simulink model "control_mimo_simulink_Clase10"  (R2019b)
settings: Solver=ode45  StartTime=0.0  StopTime=7  MaxStep=0.01  RelTol=1e-3
values from neighbouring files (symbols this model uses):
  A = [-0.005509 0 0 -0.1588 ... (first row only)    [controlador_mimo_Clase10.m]
  B = [0.28 0 -0.01348 0 ... (first row only)    [controlador_mimo_Clase10.m]
  C = [14.21 0 0 0 ... (first row only)    [controlador_mimo_Clase10.m]
  D = [0 0 0 0 ... (first row only)    [controlador_mimo_Clase10.m]
  xini = 0*[0.2; 0.3; 0; -0.2]    [controlador_mimo_Clase10.m]
undefined symbols (not defined in the file or in its folder): AL, BL, CL, DL, u10, u20, u30, x10n, x20n, x30n
libraries: cstblocks x16
settings Model: Creator=B13  LastModifiedBy=l53

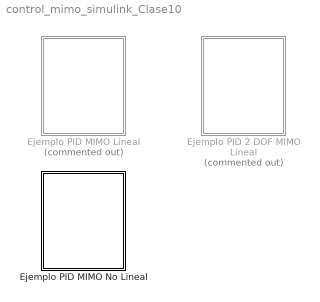
== system control_mimo_simulink_Clase10 ==
  Ejemplo PID 2 DOF MIMO Lineal : Subsystem  Commented=on
  Ejemplo PID MIMO Lineal : Subsystem  Commented=on
  Ejemplo PID MIMO No Lineal : Subsystem

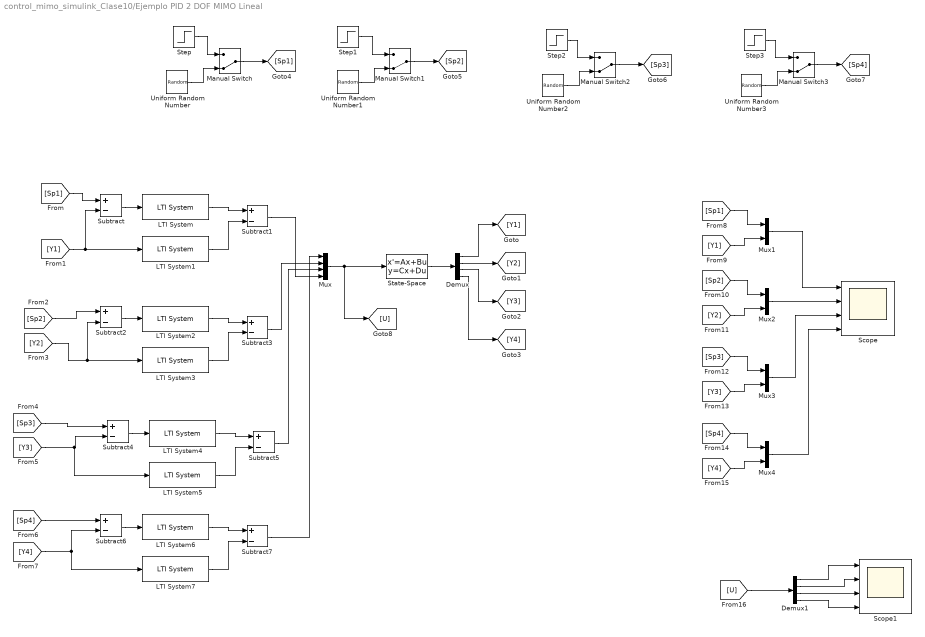
== system control_mimo_simulink_Clase10/Ejemplo PID 2 DOF MIMO Lineal ==
  Demux : Demux
  Demux1 : Demux
  LTI System : cstblocks/LTI System  sys=C14a  IC=[]
  LTI System1 : cstblocks/LTI System  sys=C14b  IC=[]
  LTI System2 : cstblocks/LTI System  sys=C22a  IC=[]
  LTI System3 : cstblocks/LTI System  sys=C22b  IC=[]
  LTI System4 : cstblocks/LTI System  sys=C33a  IC=[]
  LTI System5 : cstblocks/LTI System  sys=C33b  IC=[]
  LTI System6 : cstblocks/LTI System  sys=C41a  IC=[]
  LTI System7 : cstblocks/LTI System  sys=C41b  IC=[]
  Manual Switch{,1..3} (4 alike) : ManualSwitch  CurrentSetting=0
  Mux : Mux
  Mux{1..4} (4 alike) : Mux  Inputs=2
  Scope : Scope  NumInputPorts=4
  Scope1 : Scope  NumInputPorts=4
  State-Space : StateSpace  A=A  B=B  C=C  D=D  InitialCondition=xini
  Step : Step  Time=0  After=0  SampleTime=0
  Step1 : Step  Time=0  After=0  SampleTime=0
  Step2 : Step  Time=0  After=0  SampleTime=0
  Step3 : Step  Time=0  SampleTime=0
  Subtract{,1..7} (8 alike) : Sum  Inputs=+-
  Uniform Random Number : UniformRandomNumber  SampleTime=800
  Uniform Random Number1 : UniformRandomNumber  SampleTime=1000
  Uniform Random Number2 : UniformRandomNumber  SampleTime=1200
  Uniform Random Number3 : UniformRandomNumber  SampleTime=1500
  wires:
  Mux2/1 -> Scope/2
  Step1/1 -> Manual Switch1/1
  Manual Switch/1 -> [Sp1]
  [U] -> Demux1/1
  Step2/1 -> Manual Switch2/1
  [Sp2] -> Mux2/1
  Uniform Random Number/1 -> Manual Switch/2
  [Y3] -> Mux3/2
  Demux/4 -> [Y4]
  Mux/1 -> [U], State-Space/1
  Step3/1 -> Manual Switch3/1
  Manual Switch2/1 -> [Sp3]
  Manual Switch1/1 -> [Sp2]
  Manual Switch3/1 -> [Sp4]
  Mux3/1 -> Scope/3
  Uniform Random Number2/1 -> Manual Switch2/2
  Uniform Random Number3/1 -> Manual Switch3/2
  Uniform Random Number1/1 -> Manual Switch1/2
  Step/1 -> Manual Switch/1
  Demux/2 -> [Y2]
  [Y4] -> Mux4/2
  [Sp1] -> Mux1/1
  [Sp4] -> Mux4/1
  Demux/3 -> [Y3]
  State-Space/1 -> Demux/1
  Demux/1 -> [Y1]
  Demux1/3 -> Scope1/3
  Demux1/1 -> Scope1/1
  Demux1/4 -> Scope1/4
  [Sp3] -> Mux3/1
  [Y1] -> Mux1/2
  Mux1/1 -> Scope/1
  Mux4/1 -> Scope/4
  [Y2] -> Mux2/2
  Demux1/2 -> Scope1/2
  [Sp1] -> Subtract/1
  [Y1] -> Subtract/2, LTI System1/1
  Subtract/1 -> LTI System/1
  LTI System/1 -> Subtract1/1
  LTI System1/1 -> Subtract1/2
  Subtract1/1 -> Mux/4
  [Y2] -> Subtract2/2, LTI System3/1
  [Sp2] -> Subtract2/1
  LTI System3/1 -> Subtract3/2
  LTI System2/1 -> Subtract3/1
  Subtract2/1 -> LTI System2/1
  Subtract3/1 -> Mux/2
  [Sp3] -> Subtract4/1
  LTI System5/1 -> Subtract5/2
  LTI System4/1 -> Subtract5/1
  Subtract4/1 -> LTI System4/1
  [Y3] -> LTI System5/1, Subtract4/2
  Subtract5/1 -> Mux/3
  [Sp4] -> Subtract6/1
  LTI System7/1 -> Subtract7/2
  LTI System6/1 -> Subtract7/1
  Subtract6/1 -> LTI System6/1
  [Y4] -> Subtract6/2, LTI System7/1
  Subtract7/1 -> Mux/1

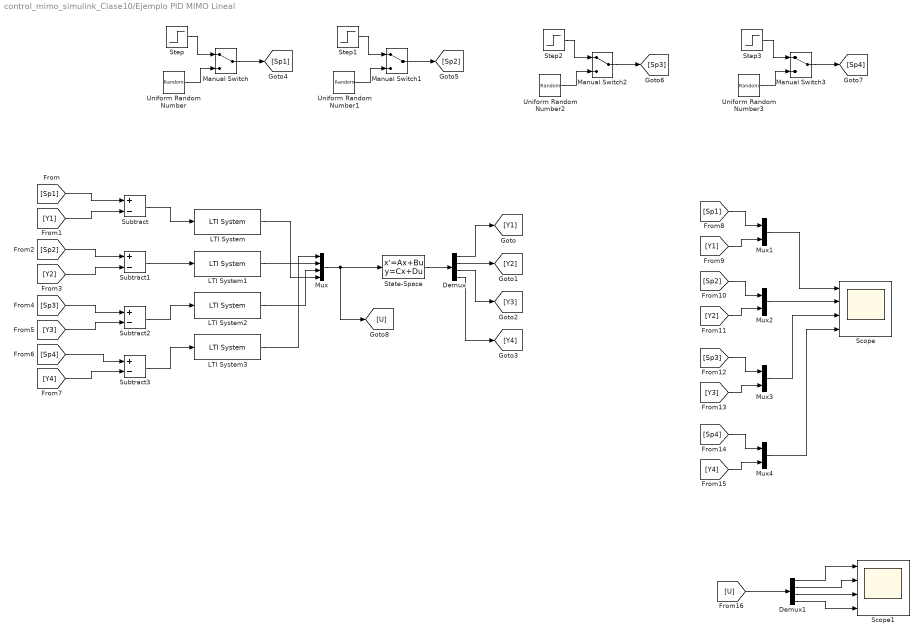
== system control_mimo_simulink_Clase10/Ejemplo PID MIMO Lineal ==
  Demux : Demux
  Demux1 : Demux
  LTI System : cstblocks/LTI System  sys=C14  IC=[]
  LTI System1 : cstblocks/LTI System  sys=C22  IC=[]
  LTI System2 : cstblocks/LTI System  sys=C33  IC=[]
  LTI System3 : cstblocks/LTI System  sys=C41  IC=[]
  Manual Switch{,1..3} (4 alike) : ManualSwitch
  Mux : Mux
  Mux{1..4} (4 alike) : Mux  Inputs=2
  Scope : Scope  NumInputPorts=4
  Scope1 : Scope  NumInputPorts=4
  State-Space : StateSpace  A=A  B=B  C=C  D=D  InitialCondition=xini
  Step{,1..3} (4 alike) : Step  Time=0  After=0  SampleTime=0
  Subtract{,1..3} (4 alike) : Sum  Inputs=+-
  Uniform Random Number : UniformRandomNumber  SampleTime=500
  Uniform Random Number1 : UniformRandomNumber  SampleTime=700
  Uniform Random Number2 : UniformRandomNumber  SampleTime=900
  Uniform Random Number3 : UniformRandomNumber  SampleTime=1100
  wires:
  Mux2/1 -> Scope/2
  Step1/1 -> Manual Switch1/1
  Manual Switch/1 -> [Sp1]
  [Y1] -> Subtract/2
  [U] -> Demux1/1
  LTI System/1 -> Mux/4
  Step2/1 -> Manual Switch2/1
  [Sp2] -> Mux2/1
  Uniform Random Number/1 -> Manual Switch/2
  [Y3] -> Mux3/2
  Demux/4 -> [Y4]
  Mux/1 -> [U], State-Space/1
  Step3/1 -> Manual Switch3/1
  Subtract2/1 -> LTI System2/1
  LTI System1/1 -> Mux/2
  Manual Switch2/1 -> [Sp3]
  Manual Switch1/1 -> [Sp2]
  Subtract3/1 -> LTI System3/1
  Manual Switch3/1 -> [Sp4]
  Mux3/1 -> Scope/3
  Subtract1/1 -> LTI System1/1
  Uniform Random Number2/1 -> Manual Switch2/2
  Uniform Random Number3/1 -> Manual Switch3/2
  Uniform Random Number1/1 -> Manual Switch1/2
  Step/1 -> Manual Switch/1
  [Y3] -> Subtract2/2
  [Sp1] -> Subtract/1
  Demux/2 -> [Y2]
  [Y4] -> Mux4/2
  [Sp1] -> Mux1/1
  LTI System2/1 -> Mux/3
  [Sp4] -> Mux4/1
  [Y2] -> Subtract1/2
  [Sp2] -> Subtract1/1
  Demux/3 -> [Y3]
  [Sp3] -> Subtract2/1
  Subtract/1 -> LTI System/1
  [Sp4] -> Subtract3/1
  State-Space/1 -> Demux/1
  LTI System3/1 -> Mux/1
  [Y4] -> Subtract3/2
  Demux/1 -> [Y1]
  Demux1/3 -> Scope1/3
  Demux1/1 -> Scope1/1
  Demux1/4 -> Scope1/4
  [Sp3] -> Mux3/1
  [Y1] -> Mux1/2
  Mux1/1 -> Scope/1
  Mux4/1 -> Scope/4
  [Y2] -> Mux2/2
  Demux1/2 -> Scope1/2

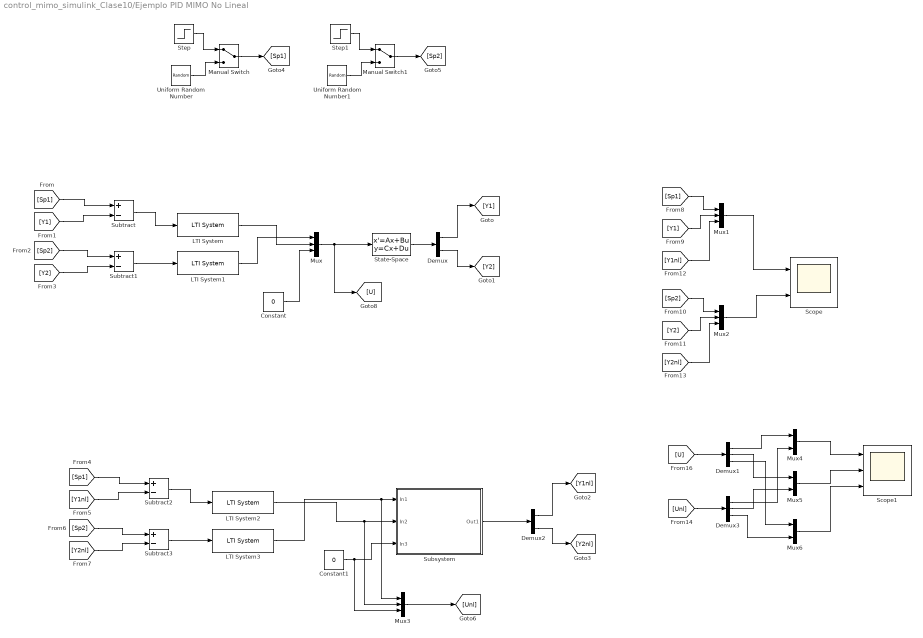
== system control_mimo_simulink_Clase10/Ejemplo PID MIMO No Lineal ==
  Constant : Constant  Value=0
  Constant1 : Constant  Value=0
  Demux : Demux  Outputs=2
  Demux1 : Demux  Outputs=3
  Demux2 : Demux  Outputs=2
  Demux3 : Demux  Outputs=3
  LTI System : cstblocks/LTI System  sys=C12  IC=[]
  LTI System1 : cstblocks/LTI System  sys=C21  IC=[]
  LTI System2 : cstblocks/LTI System  sys=C12  IC=[]
  LTI System3 : cstblocks/LTI System  sys=C21  IC=[]
  Manual Switch : ManualSwitch
  Manual Switch1 : ManualSwitch
  Mux{,1..3} (4 alike) : Mux  Inputs=3
  Mux4 : Mux  Inputs=2
  Mux5 : Mux  Inputs=2
  Mux6 : Mux  Inputs=2
  Scope : Scope  NumInputPorts=2
  Scope1 : Scope  NumInputPorts=3
  State-Space : StateSpace  A=AL  B=BL  C=CL  D=DL  InitialCondition=xini
  Step : Step  Time=0  After=0  SampleTime=0
  Step1 : Step  Time=0  After=0  SampleTime=0
  Subsystem : Subsystem
  Subtract{,1..3} (4 alike) : Sum  Inputs=+-
  Uniform Random Number : UniformRandomNumber  Minimum=-5  Maximum=5  SampleTime=4
  Uniform Random Number1 : UniformRandomNumber  Minimum=-5  Maximum=5  SampleTime=6
  wires:
  Mux2/1 -> Scope/2
  Step1/1 -> Manual Switch1/1
  Manual Switch/1 -> [Sp1]
  [Y1] -> Subtract/2
  [U] -> Demux1/1
  [Sp2] -> Mux2/1
  Uniform Random Number/1 -> Manual Switch/2
  Mux/1 -> [U], State-Space/1
  Manual Switch1/1 -> [Sp2]
  Subtract1/1 -> LTI System1/1
  Uniform Random Number1/1 -> Manual Switch1/2
  Step/1 -> Manual Switch/1
  [Sp1] -> Subtract/1
  Demux/2 -> [Y2]
  [Sp1] -> Mux1/1
  [Y2] -> Subtract1/2
  [Sp2] -> Subtract1/1
  Subtract/1 -> LTI System/1
  State-Space/1 -> Demux/1
  Demux/1 -> [Y1]
  [Y1] -> Mux1/2
  Mux1/1 -> Scope/1
  [Y2] -> Mux2/2
  LTI System/1 -> Mux/2
  LTI System1/1 -> Mux/1
  Constant/1 -> Mux/3
  [Y1nl] -> Subtract2/2
  Demux2/1 -> [Y1nl]
  [Sp2] -> Subtract3/1
  Subtract2/1 -> LTI System2/1
  Demux2/2 -> [Y2nl]
  [Sp1] -> Subtract2/1
  [Y2nl] -> Subtract3/2
  Subtract3/1 -> LTI System3/1
  LTI System2/1 -> Mux3/2, Subsystem/2(In2)
  LTI System3/1 -> Mux3/1, Subsystem/1(In1)
  Constant1/1 -> Mux3/3, Subsystem/3(In3)
  Mux3/1 -> [Unl]
  Subsystem/1(Out1) -> Demux2/1
  [Y1nl] -> Mux1/3
  [Y2nl] -> Mux2/3
  [Unl] -> Demux3/1
  Mux4/1 -> Scope1/1
  Demux1/1 -> Mux4/1
  Demux3/1 -> Mux4/2
  Demux1/2 -> Mux5/1
  Demux3/2 -> Mux5/2
  Demux1/3 -> Mux6/1
  Demux3/3 -> Mux6/2
  Mux6/1 -> Scope1/3
  Mux5/1 -> Scope1/2

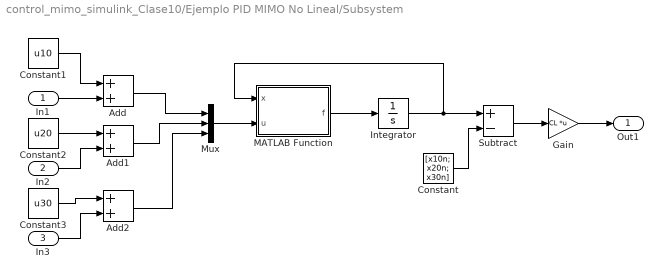
== system control_mimo_simulink_Clase10/Ejemplo PID MIMO No Lineal/Subsystem ==
  In1 : Inport
  In2 : Inport  Port=2
  In3 : Inport  Port=3
  Add : Sum
  Add1 : Sum
  Add2 : Sum
  Constant : Constant  Value=[x10n; x20n; x30n]
  Constant1 : Constant  Value=u10
  Constant2 : Constant  Value=u20
  Constant3 : Constant  Value=u30
  Gain : Gain  Gain=CL  Multiplication=Matrix(K*u)
  Integrator : Integrator  InitialCondition=[x10n; x20n; x30n] + xini
  MATLAB Function : MATLAB Function  TreatAsAtomicUnit=on
  Mux : Mux  Inputs=3
  Subtract : Sum  Inputs=+-
  Out1 : Outport
  wires:
  MATLAB Function/1(f) -> Integrator/1
  Integrator/1 -> Subtract/1, MATLAB Function/1(x)
  Subtract/1 -> Gain/1
  Constant/1 -> Subtract/2
  Gain/1 -> Out1/1
  Mux/1 -> MATLAB Function/2(u)
  Add/1 -> Mux/1
  In1/1 -> Add/2
  Add1/1 -> Mux/2
  Add2/1 -> Mux/3
  Constant1/1 -> Add/1
  Constant2/1 -> Add1/1
  In2/1 -> Add1/2
  Constant3/1 -> Add2/1
  In3/1 -> Add2/2

== matlab function control_mimo_simulink_Clase10/Ejemplo PID MIMO No Lineal/Subsystem/MATLAB Function ==
  data: x input; u input; f output
function f = fcn(x,u)

x1 = x(1);
x2 = x(2);
x3 = x(3);
u1 = u(1);
u2 = u(2);
u3 = u(3);
a = 1;
b = 1;
c = 1;
f1 = -a*x1^2 + x2 +u2*u3;
f2 = -x2 + b*x3 - u1*u3;
f3 = -c*x3^2 + exp(-u1);
f = [f1;f2;f3];
